simulink library "Robust_MPC_Library"  (R2013a)
settings: Solver=ode45  StartTime=0.0  StopTime=10.0  RelTol=1e-3
undefined symbols (not defined in the file): add_usys_d, exp_sol_x_mp, sol_x_mp, sol_x_mp_Fi, sol_x_mp_Gi, sol_x_mp_Pn
settings Model: Creator=Kostas  LastModifiedBy=Kostas

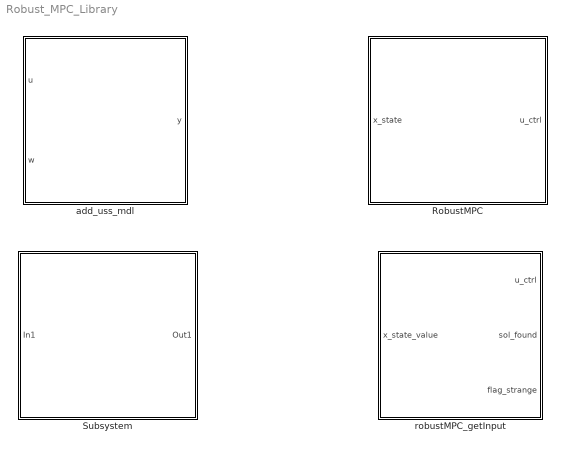
== system Robust_MPC_Library ==
  RobustMPC : Subsystem
  Subsystem : Subsystem
  add_uss_mdl : Subsystem  mask{add_usys_d_struct=add_usys_d}
      mask prompts: add_usys_d_struct "Provide Additive Uncertainty Structure"
  robustMPC_getInput : Subsystem

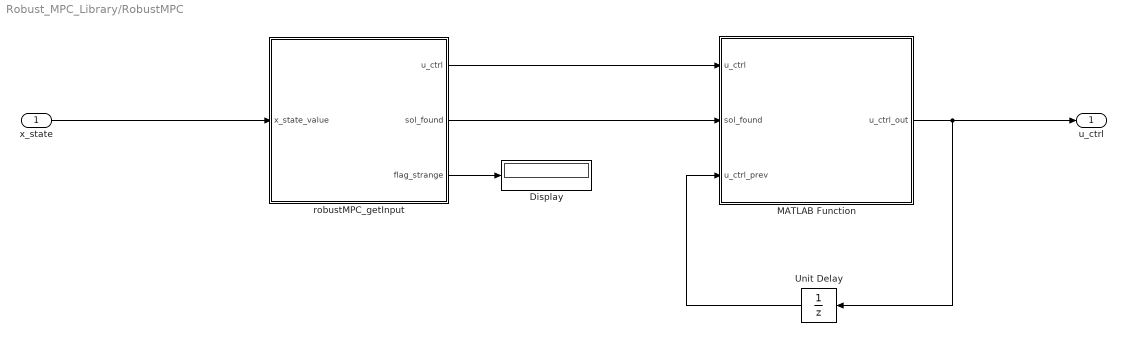
== system Robust_MPC_Library/RobustMPC ==
  x_state : Inport
  Display : Display
  MATLAB Function : MATLAB Function  TreatAsAtomicUnit=on
  Unit Delay : UnitDelay  SampleTime=-1
  robustMPC_getInput : Subsystem  mask{exp_sol_x_mp=exp_sol_x_mp}
      mask prompts: exp_sol_x_mp "Provide Robust MPC Multiparametric Solution"
  u_ctrl : Outport
  wires:
  x_state/1 -> robustMPC_getInput/1(x_state_value)
  robustMPC_getInput/1(u_ctrl) -> MATLAB Function/1(u_ctrl)
  robustMPC_getInput/2(sol_found) -> MATLAB Function/2(sol_found)
  MATLAB Function/1(u_ctrl_out) -> Unit Delay/1, u_ctrl/1
  Unit Delay/1 -> MATLAB Function/3(u_ctrl_prev)
  robustMPC_getInput/3(flag_strange) -> Display/1

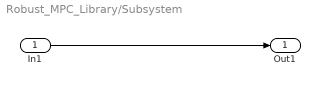
== system Robust_MPC_Library/Subsystem ==
  In1 : Inport
  Out1 : Outport
  wires:
  In1/1 -> Out1/1

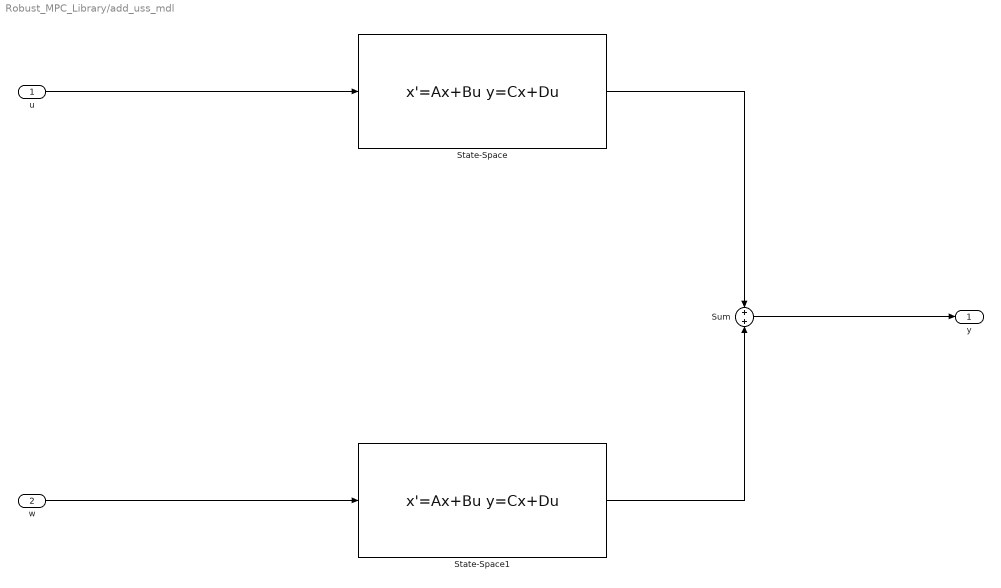
== system Robust_MPC_Library/add_uss_mdl ==
  u : Inport
  w : Inport  Port=2
  State-Space : StateSpace  A=add_usys_d_struct.continuous.matrices.A  B=add_usys_d_struct.continuous.matrices.B  C=add_usys_d_struct.continuous.matrices.C  D=add_usys_d_struct.continuous.matrices.D
  State-Space1 : StateSpace  A=add_usys_d_struct.continuous.matrices.A  B=add_usys_d_struct.continuous.matrices.E  C=add_usys_d_struct.continuous.matrices.C  D=add_usys_d_struct.continuous.matrices.D
  Sum : Sum  Inputs=+|+
  y : Outport
  wires:
  u/1 -> State-Space/1
  w/1 -> State-Space1/1
  State-Space/1 -> Sum/1
  State-Space1/1 -> Sum/2
  Sum/1 -> y/1

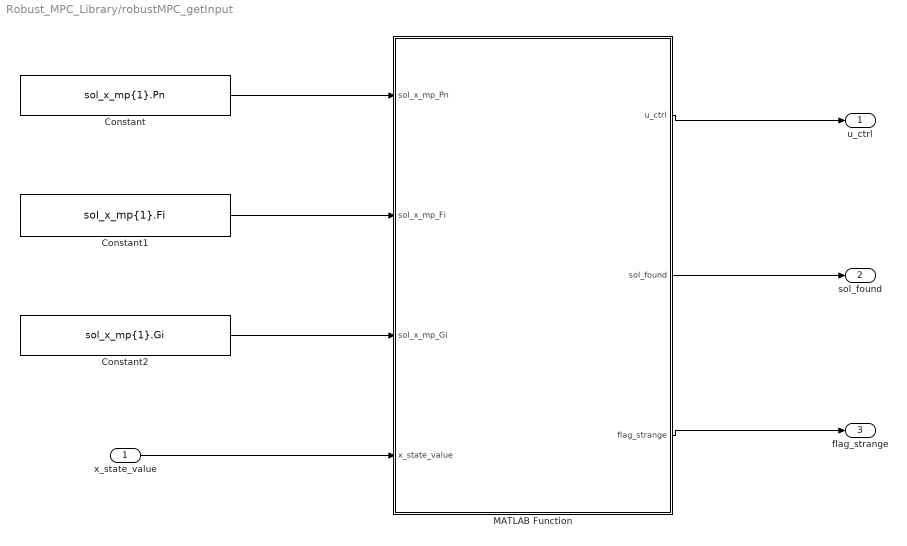
== system Robust_MPC_Library/robustMPC_getInput ==
  x_state_value : Inport
  Constant : Constant  Value=sol_x_mp{1}.Pn
  Constant1 : Constant  Value=sol_x_mp{1}.Fi
  Constant2 : Constant  Value=sol_x_mp{1}.Gi
  MATLAB Function : MATLAB Function  TreatAsAtomicUnit=on
  u_ctrl : Outport
  sol_found : Outport  Port=2
  flag_strange : Outport  Port=3
  wires:
  Constant/1 -> MATLAB Function/1(sol_x_mp_Pn)
  Constant1/1 -> MATLAB Function/2(sol_x_mp_Fi)
  Constant2/1 -> MATLAB Function/3(sol_x_mp_Gi)
  x_state_value/1 -> MATLAB Function/4(x_state_value)
  MATLAB Function/1(u_ctrl) -> u_ctrl/1
  MATLAB Function/2(sol_found) -> sol_found/1
  MATLAB Function/3(flag_strange) -> flag_strange/1

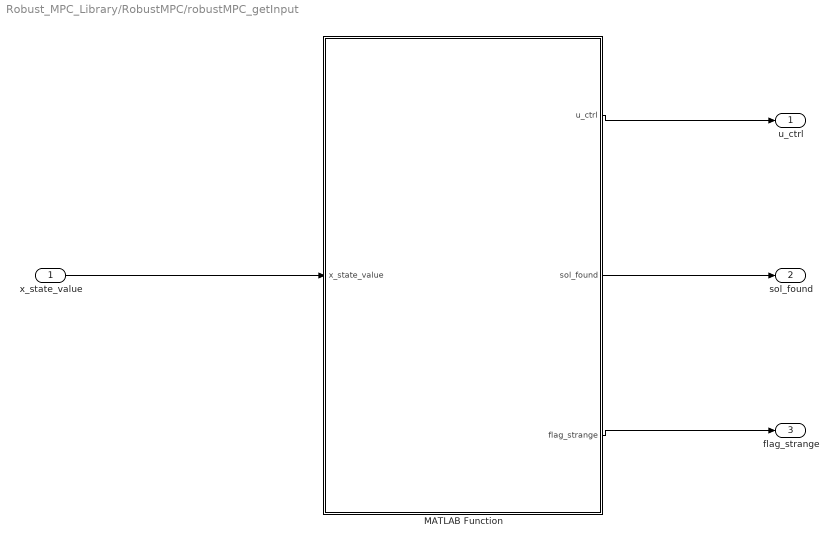
== system Robust_MPC_Library/RobustMPC/robustMPC_getInput ==
  x_state_value : Inport
  MATLAB Function : MATLAB Function  TreatAsAtomicUnit=on
  u_ctrl : Outport
  sol_found : Outport  Port=2
  flag_strange : Outport  Port=3
  wires:
  x_state_value/1 -> MATLAB Function/1(x_state_value)
  MATLAB Function/1(u_ctrl) -> u_ctrl/1
  MATLAB Function/2(sol_found) -> sol_found/1
  MATLAB Function/3(flag_strange) -> flag_strange/1

== matlab function Robust_MPC_Library/RobustMPC/MATLAB Function ==
  data: u_ctrl input; sol_found input; u_ctrl_out output; u_ctrl_prev input
function u_ctrl_out = safety_ctrl(u_ctrl,sol_found,u_ctrl_prev)
%#codegen

u_ctrl_out = u_ctrl;

if((sol_found == 0))
    u_ctrl = u_ctrl_prev;
end

end

== matlab function Robust_MPC_Library/robustMPC_getInput/MATLAB Function ==
  data: sol_x_mp_Pn input; sol_x_mp_Fi input; sol_x_mp_Gi input; u_ctrl output; x_state_value input; sol_found output; flag_strange output
function [u_ctrl,sol_found, flag_strange] = robustmpc_getInput(sol_x_mp_Pn, sol_x_mp_Fi,sol_x_mp_Gi,x_state_value)
%
%   get control action from the explicit robust mpc computed using YALMIP
%
%   Syntax:
%   [u_ctrl,sol_found] = robustmpc_getInput(sol_x_mp, x_state_value)
%
%   Inputs:
%   sol_x_mp        : Multiparametric Robust MPC explicit solution
%   x_state_value   : value of the state vector
%
%   Outputs:
%   u_ctrl          : control action
%   sol_found       : flag indicating whether a solution was found
%
%   Authors: Kostas Alexis (konstantinos.alexis@mavt.ethz.ch)

sol_found = 1;
[i,j] = isinside(sol_x_mp_Pn, x_state_value);

flag_strange = 0;
if(length(j)>1)
    j = j(1); % this requires further analysis
    flag_strange = 1;
end

if(isempty(j)==0)
    u_ctrl = sol_x_mp_Fi{j}*x_state_value + sol_x_mp_Gi{j};
    sol_found = 1;
else
    sol_found = 0;
    u_ctrl = NaN;
end

if(flag_strange == 1)
    u_ctrl = 0.0256;
end
end

== matlab function Robust_MPC_Library/RobustMPC/robustMPC_getInput/MATLAB Function ==
  data: sol_x_mp_Pn parameter; sol_x_mp_Fi parameter; sol_x_mp_Gi parameter; u_ctrl output; x_state_value input; sol_found output; flag_strange output
function [u_ctrl,sol_found, flag_strange] = robustmpc_getInput(sol_x_mp_Pn, sol_x_mp_Fi,sol_x_mp_Gi,x_state_value)
%
%   get control action from the explicit robust mpc computed using YALMIP
%
%   Syntax:
%   [u_ctrl,sol_found] = robustmpc_getInput(sol_x_mp, x_state_value)
%
%   Inputs:
%   sol_x_mp        : Multiparametric Robust MPC explicit solution
%   x_state_value   : value of the state vector
%
%   Outputs:
%   u_ctrl          : control action
%   sol_found       : flag indicating whether a solution was found
%
%   Authors: Kostas Alexis (konstantinos.alexis@mavt.ethz.ch)

sol_found = 1;
[i,j] = isinside(sol_x_mp_Pn, x_state_value);

flag_strange = 0;
if(length(j)>1)
    j = j(1); % this requires further analysis
    flag_strange = 1;
end

if(isempty(j)==0)
    u_ctrl = sol_x_mp_Fi{j}*x_state_value + sol_x_mp_Gi{j};
    sol_found = 1;
else
    sol_found = 0;
    u_ctrl = NaN;
end

if(flag_strange == 1)
    u_ctrl = 0.0256;
end
end
